simulink model "example_InputFluid"  (Simulink 8.2)
settings: Solver=VariableStepDiscrete  StartTime=0.0  StopTime=10.0  MaxStep=0.2  RelTol=1e-3
libraries: carnot x2
settings Model: Creator=drhf  LastModifiedBy=drhf

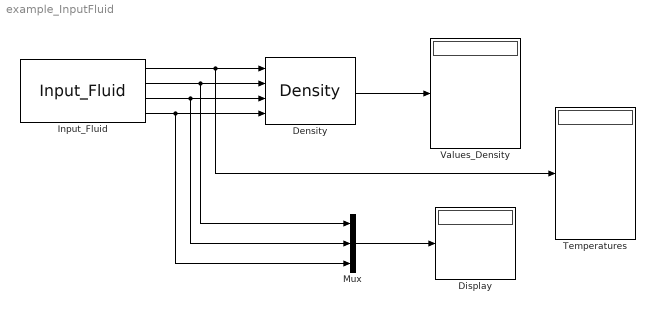
== system example_InputFluid ==
  Density : carnot/Basic/Material_Properties/Density  VariantControl=CarlibClassic  INPUTARGUMENTS=state variables (classic)  DEBUGLEVEL=DEBUGLEVEL  MAXTOTALWARNINGS=inf  MAXCONSECUTIVEWARNINGS=inf  WRITETOFILE=0  FILENAME='errors.txt'
  Display : Display
  Input_Fluid : carnot/Basic/Material_Properties/Input_Fluid  fluid=Water  T=[10:10:50]  p=1e5  x=0.005
  Mux : Mux  Inputs=3
  Temperatures : Display
  Values_Density : Display
  wires:
  Input_Fluid/1 -> Density/1, Temperatures/1
  Input_Fluid/2 -> Density/2, Mux/1
  Input_Fluid/3 -> Density/3, Mux/2
  Input_Fluid/4 -> Density/4, Mux/3
  Density/1 -> Values_Density/1
  Mux/1 -> Display/1
